simulink model "rRegenPaddle"  (R2024b)
settings: Solver=FixedStepDiscrete  StartTime=0.0  StopTime=1  FixedStep=0.001  RelTol=1e-3  EnableMultiTasking=on
undefined symbols (not defined in the file): rRegenPaddleOverlapThreshold, rRegenSensorGain
libraries: simulink x1
settings Model: DataDictionary=Master_Dictionary.sldd  EnableAccessToBaseWorkspace=off  Creator=torni  LastModifiedBy=oxbro
settings SolverCC: AlgebraicLoopSolver=TrustRegion
settings DataIOCC: ReturnWorkspaceOutputs=off
settings OptimizationCC: DefaultParameterBehavior=Inlined  EnhancedBackFolding=on  PassReuseOutputArgsAs=Individual arguments  ZeroExternalMemoryAtStartup=off  ZeroInternalMemoryAtStartup=off  MaxStackSize=512  OptimizeBlockOrder=speed  DifferentSizesBufferReuse=on  OptimizationCustomize=off  EfficientTunableParamExpr=on
settings DebuggingCC: ParameterTunabilityLossMsg=error  UnconnectedInputMsg=warning  UnconnectedOutputMsg=warning  UnconnectedLineMsg=warning  ArithmeticOperatorsInVariantConditions=warning
settings HardwareCC: ProdBitPerPointer=32  ProdBitPerSizeT=32  ProdBitPerPtrDiffT=32  ProdLargestAtomicInteger=Long  ProdLargestAtomicFloat=Double  ProdWordSize=32  ProdLongLongMode=on  ProdHWDeviceType=ARM Compatible->ARM Cortex-M
settings ModelReferenceCC: EnableRefExpFcnMdlSchedulingChecks=on
settings SFSimCC: MATLABDynamicMemAlloc=off  CustomCodeUndefinedFunction=UseInterfaceOnly
settings RTWCC: Description=Embedded Coder  SystemTargetFile=ert.tlc  HardwareBoard=STM32H7xx Based (Single-core)  TemplateMakefile=ert_default_tmf  CustomHeaderCode="#include \"stm32h7xx_ll_tim.h\""  CustomInitializer=LL_TIM_EnableCounter(TIM2);  Toolchain=GNU Tools for ARM Embedded Processors  GPUComputeCapability=3.5
settings CodeAppCC: ForceParamTrailComments=on  IgnoreCustomStorageClasses=off  OperatorAnnotations=on  SimulinkDataObjDesc=on  SFDataObjDesc=on  InsertBlockDesc=on
settings ERTTargetCC: TargetLangStandard=C99 (ISO)  CodeReplacementLibrary=ARM Cortex-M  ExtModeTransport=3  ExtModeStaticAlloc=on  ExtModeStaticAllocSize=2048  ExtModeMexFile=ext_xcp  ExtModeIntrfLevel=Level2 - Open

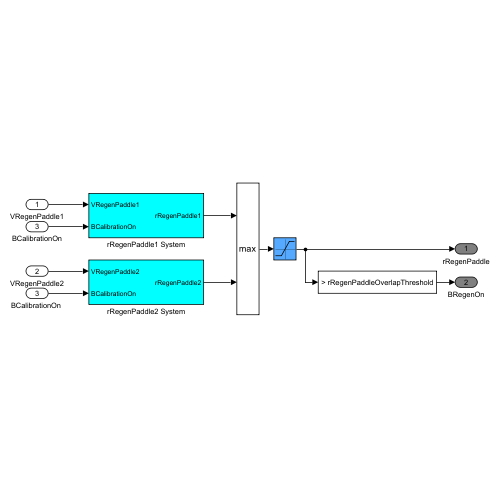
[thumbnail: Simulink's stored preview of the top-level diagram]
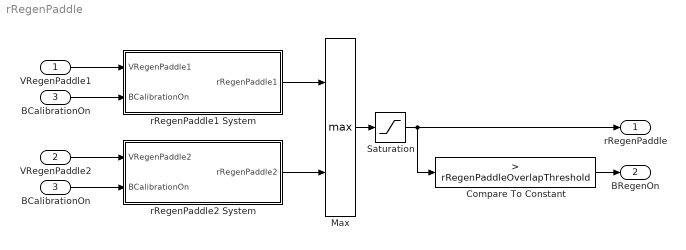
== system rRegenPaddle ==
  VRegenPaddle1 : Inport  OutDataTypeStr=double
  VRegenPaddle2 : Inport  Port=2  OutDataTypeStr=double
  BCalibrationOn : Inport  Port=3  OutDataTypeStr=boolean
  "BCalibrationOn " : InportShadow  Port=3  OutDataTypeStr=boolean
  Compare To Constant : simulink/Logic and Bit Operations/Compare To Constant  relop=>  const=rRegenPaddleOverlapThreshold  OutDataTypeStr=boolean
  Max : MinMax  Function=max  Inputs=2
  Saturation : Saturate  UpperLimit=100  LowerLimit=0
  rRegenPaddle1 System : Subsystem
  rRegenPaddle2 System : Subsystem
  rRegenPaddle : Outport  OutDataTypeStr=double  VectorParamsAs1DForOutWhenUnconnected=off
  "BRegenOn " : Outport  Port=2  OutDataTypeStr=boolean  VectorParamsAs1DForOutWhenUnconnected=off
  wires:
  Saturation/1 -> rRegenPaddle/1, Compare To Constant/1
  Compare To Constant/1 -> "BRegenOn "/1
  Max/1 -> Saturation/1
  VRegenPaddle2/1 -> rRegenPaddle2 System/1(VRegenPaddle2)
  VRegenPaddle1/1 -> rRegenPaddle1 System/1(VRegenPaddle1)
  rRegenPaddle2 System/1(rRegenPaddle2) -> Max/2
  rRegenPaddle1 System/1(rRegenPaddle1) -> Max/1
  "BCalibrationOn "/1 -> rRegenPaddle2 System/2(BCalibrationOn)
  BCalibrationOn/1 -> rRegenPaddle1 System/2(BCalibrationOn)

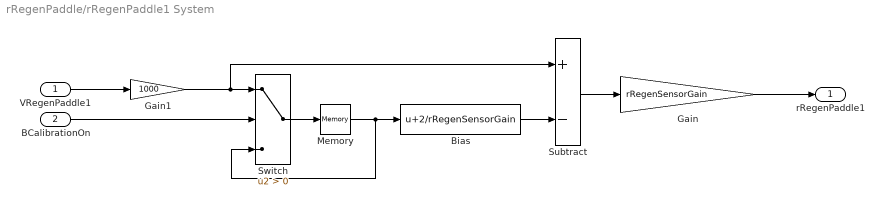
== system rRegenPaddle/rRegenPaddle1 System ==
  VRegenPaddle1 : Inport  OutDataTypeStr=double
  BCalibrationOn : Inport  Port=2  OutDataTypeStr=boolean
  Bias : Bias  Bias=2/rRegenSensorGain  SaturateOnIntegerOverflow=off
  Gain : Gain  Gain=rRegenSensorGain
  Gain1 : Gain  Gain=1000
  Memory : Memory  InitialCondition=300  InheritSampleTime=on
  Subtract : Sum  Inputs=+-
  Switch : Switch  Criteria=u2 > Threshold  SaturateOnIntegerOverflow=off  InputSameDT=off
  rRegenPaddle1 : Outport  OutDataTypeStr=double  VectorParamsAs1DForOutWhenUnconnected=off
  wires:
  BCalibrationOn/1 -> Switch/2
  VRegenPaddle1/1 -> Gain1/1
  Switch/1 -> Memory/1
  Memory/1 -> Switch/3, Bias/1
  Bias/1 -> Subtract/2
  Subtract/1 -> Gain/1
  Gain/1 -> rRegenPaddle1/1
  Gain1/1 -> Subtract/1, Switch/1

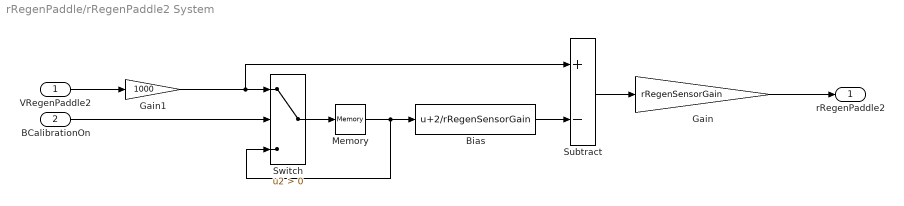
== system rRegenPaddle/rRegenPaddle2 System ==
  VRegenPaddle2 : Inport  OutDataTypeStr=double
  BCalibrationOn : Inport  Port=2  OutDataTypeStr=boolean
  Bias : Bias  Bias=2/rRegenSensorGain  SaturateOnIntegerOverflow=off
  Gain : Gain  Gain=rRegenSensorGain
  Gain1 : Gain  Gain=1000
  Memory : Memory  InitialCondition=300  InheritSampleTime=on
  Subtract : Sum  Inputs=+-
  Switch : Switch  Criteria=u2 > Threshold  SaturateOnIntegerOverflow=off  InputSameDT=off
  rRegenPaddle2 : Outport  OutDataTypeStr=double  VectorParamsAs1DForOutWhenUnconnected=off
  wires:
  Gain/1 -> rRegenPaddle2/1
  Bias/1 -> Subtract/2
  VRegenPaddle2/1 -> Gain1/1
  Switch/1 -> Memory/1
  Memory/1 -> Switch/3, Bias/1
  BCalibrationOn/1 -> Switch/2
  Subtract/1 -> Gain/1
  Gain1/1 -> Subtract/1, Switch/1
